simulink model "TST_AirCtl_Co"  (R2016b)
settings: Solver=FixedStepDiscrete  StartTime=0.0  StopTime=simTime  FixedStep=sampleTime  RelTol=1e-3
values from neighbouring files (symbols this model uses):
  testCase = 1    [initTST_AirCtl_Co_001.m]    (also in initTST_AirCtl_Co_002.m = 2)
libraries: simulink x19, UnitTest_Lib x16
settings Model: Creator=zhulinfeng  LastModifiedBy=zhulinfeng
settings DebuggingCC: SignalRangeChecking=error

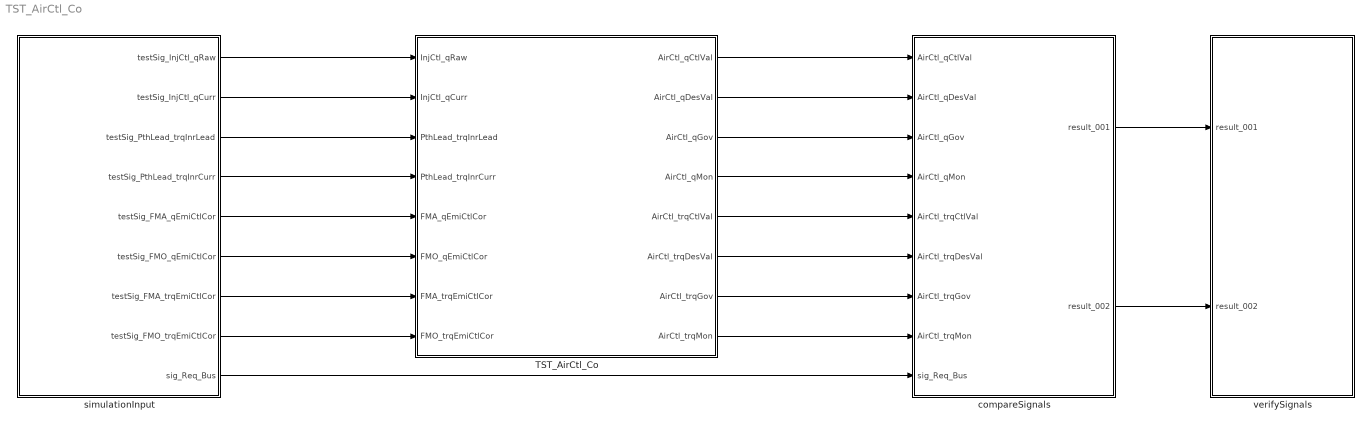
== system TST_AirCtl_Co ==
  TST_AirCtl_Co : Subsystem
  compareSignals : Subsystem
  simulationInput : Subsystem
  verifySignals : Subsystem
  wires:
  simulationInput/1(testSig_InjCtl_qRaw) -> TST_AirCtl_Co/1(InjCtl_qRaw)
  simulationInput/2(testSig_InjCtl_qCurr) -> TST_AirCtl_Co/2(InjCtl_qCurr)
  simulationInput/3(testSig_PthLead_trqInrLead) -> TST_AirCtl_Co/3(PthLead_trqInrLead)
  simulationInput/4(testSig_PthLead_trqInrCurr) -> TST_AirCtl_Co/4(PthLead_trqInrCurr)
  simulationInput/5(testSig_FMA_qEmiCtlCor) -> TST_AirCtl_Co/5(FMA_qEmiCtlCor)
  simulationInput/6(testSig_FMO_qEmiCtlCor) -> TST_AirCtl_Co/6(FMO_qEmiCtlCor)
  simulationInput/7(testSig_FMA_trqEmiCtlCor) -> TST_AirCtl_Co/7(FMA_trqEmiCtlCor)
  simulationInput/8(testSig_FMO_trqEmiCtlCor) -> TST_AirCtl_Co/8(FMO_trqEmiCtlCor)
  TST_AirCtl_Co/1(AirCtl_qCtlVal) -> compareSignals/1(AirCtl_qCtlVal)
  TST_AirCtl_Co/2(AirCtl_qDesVal) -> compareSignals/2(AirCtl_qDesVal)
  TST_AirCtl_Co/3(AirCtl_qGov) -> compareSignals/3(AirCtl_qGov)
  TST_AirCtl_Co/4(AirCtl_qMon) -> compareSignals/4(AirCtl_qMon)
  TST_AirCtl_Co/5(AirCtl_trqCtlVal) -> compareSignals/5(AirCtl_trqCtlVal)
  TST_AirCtl_Co/6(AirCtl_trqDesVal) -> compareSignals/6(AirCtl_trqDesVal)
  TST_AirCtl_Co/7(AirCtl_trqGov) -> compareSignals/7(AirCtl_trqGov)
  TST_AirCtl_Co/8(AirCtl_trqMon) -> compareSignals/8(AirCtl_trqMon)
  simulationInput/9(sig_Req_Bus) -> compareSignals/9(sig_Req_Bus)
  compareSignals/1(result_001) -> verifySignals/1(result_001)
  compareSignals/2(result_002) -> verifySignals/2(result_002)

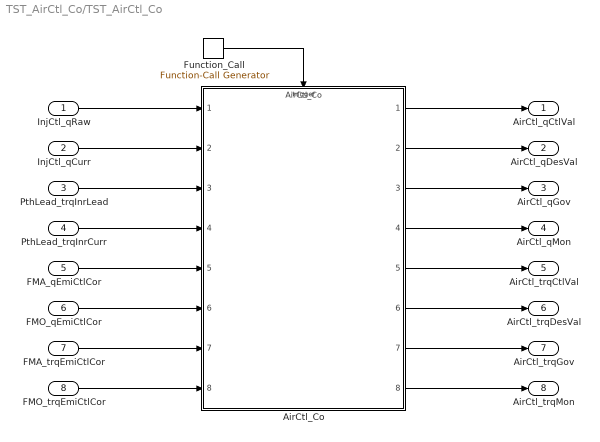
== system TST_AirCtl_Co/TST_AirCtl_Co ==
  InjCtl_qRaw : Inport
  InjCtl_qCurr : Inport  Port=2
  PthLead_trqInrLead : Inport  Port=3
  PthLead_trqInrCurr : Inport  Port=4
  FMA_qEmiCtlCor : Inport  Port=5
  FMO_qEmiCtlCor : Inport  Port=6
  FMA_trqEmiCtlCor : Inport  Port=7
  FMO_trqEmiCtlCor : Inport  Port=8
  AirCtl_Co : ModelReference  ModelNameDialog=AirCtl_Co  SimulationMode=Normal  ModelReferenceVersion=1.15  TriggerPortName=function  TriggerPortTriggerType=function-call  TriggerPortStatesWhenEnabling=held
  Function_Call : simulink/Ports & Subsystems/Function-Call Generator  sample_time=sampleTime  numberOfIterations=1
  AirCtl_qCtlVal : Outport
  AirCtl_qDesVal : Outport  Port=2
  AirCtl_qGov : Outport  Port=3
  AirCtl_qMon : Outport  Port=4
  AirCtl_trqCtlVal : Outport  Port=5
  AirCtl_trqDesVal : Outport  Port=6
  AirCtl_trqGov : Outport  Port=7
  AirCtl_trqMon : Outport  Port=8
  wires:
  Function_Call/1 -> AirCtl_Co/Trigger
  InjCtl_qRaw/1 -> AirCtl_Co/1
  InjCtl_qCurr/1 -> AirCtl_Co/2
  PthLead_trqInrLead/1 -> AirCtl_Co/3
  PthLead_trqInrCurr/1 -> AirCtl_Co/4
  FMA_qEmiCtlCor/1 -> AirCtl_Co/5
  FMO_qEmiCtlCor/1 -> AirCtl_Co/6
  FMA_trqEmiCtlCor/1 -> AirCtl_Co/7
  FMO_trqEmiCtlCor/1 -> AirCtl_Co/8
  AirCtl_Co/1 -> AirCtl_qCtlVal/1
  AirCtl_Co/2 -> AirCtl_qDesVal/1
  AirCtl_Co/3 -> AirCtl_qGov/1
  AirCtl_Co/4 -> AirCtl_qMon/1
  AirCtl_Co/5 -> AirCtl_trqCtlVal/1
  AirCtl_Co/6 -> AirCtl_trqDesVal/1
  AirCtl_Co/7 -> AirCtl_trqGov/1
  AirCtl_Co/8 -> AirCtl_trqMon/1

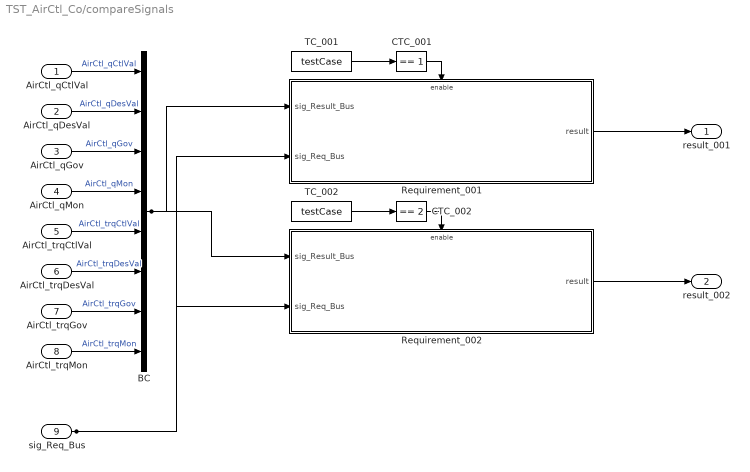
== system TST_AirCtl_Co/compareSignals ==
  AirCtl_qCtlVal : Inport
  AirCtl_qDesVal : Inport  Port=2
  AirCtl_qGov : Inport  Port=3
  AirCtl_qMon : Inport  Port=4
  AirCtl_trqCtlVal : Inport  Port=5
  AirCtl_trqDesVal : Inport  Port=6
  AirCtl_trqGov : Inport  Port=7
  AirCtl_trqMon : Inport  Port=8
  sig_Req_Bus : Inport  Port=9
  BC : BusCreator  Inputs=8
  CTC_001 : simulink/Logic and Bit Operations/Compare To Constant  relop===  const=1  OutDataTypeStr=boolean
  CTC_002 : simulink/Logic and Bit Operations/Compare To Constant  relop===  const=2  OutDataTypeStr=boolean
  Requirement_001 : Subsystem
  Requirement_002 : Subsystem
  TC_001 : Constant  Value=testCase
  TC_002 : Constant  Value=testCase
  result_001 : Outport
  result_002 : Outport  Port=2
  wires:
  AirCtl_qCtlVal/1 -> BC/1  "AirCtl_qCtlVal"
  AirCtl_qDesVal/1 -> BC/2  "AirCtl_qDesVal"
  AirCtl_qGov/1 -> BC/3  "AirCtl_qGov"
  AirCtl_qMon/1 -> BC/4  "AirCtl_qMon"
  AirCtl_trqCtlVal/1 -> BC/5  "AirCtl_trqCtlVal"
  AirCtl_trqDesVal/1 -> BC/6  "AirCtl_trqDesVal"
  AirCtl_trqGov/1 -> BC/7  "AirCtl_trqGov"
  AirCtl_trqMon/1 -> BC/8  "AirCtl_trqMon"
  TC_001/1 -> CTC_001/1
  CTC_001/1 -> Requirement_001/Enable
  sig_Req_Bus/1 -> Requirement_001/2(sig_Req_Bus), Requirement_002/2(sig_Req_Bus)
  BC/1 -> Requirement_001/1(sig_Result_Bus), Requirement_002/1(sig_Result_Bus)
  Requirement_001/1(result) -> result_001/1
  TC_002/1 -> CTC_002/1
  CTC_002/1 -> Requirement_002/Enable
  Requirement_002/1(result) -> result_002/1

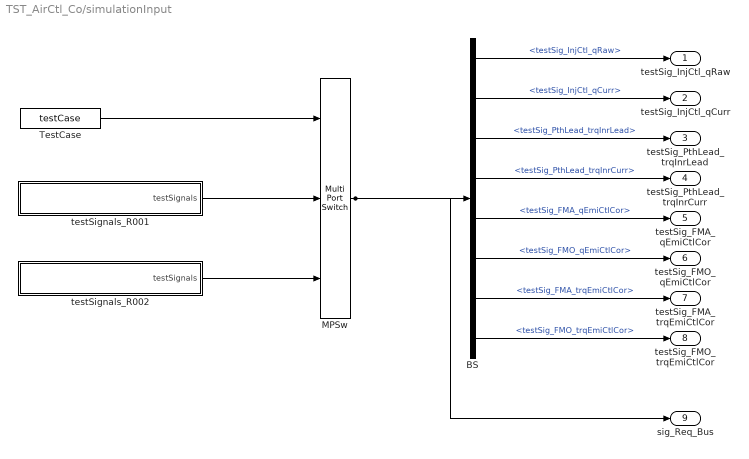
== system TST_AirCtl_Co/simulationInput ==
  BS : BusSelector  OutputSignals=testSig_InjCtl_qRaw,testSig_InjCtl_qCurr,testSig_PthLead_trqInrLead,testSig_PthLead_trqInrCurr,testSig_FMA_qEmiCtlCor,testSig_FMO_qEmiCtlCor,testSig_FMA_trqEmiCtlCor,testSig_FMO_trqEmiCtlCor
  MPSw : MultiPortSwitch  Inputs=2  SaturateOnIntegerOverflow=on  InputSameDT=on
  TestCase : Constant  Value=testCase
  testSignals_R001 : Subsystem
  testSignals_R002 : Subsystem
  testSig_InjCtl_qRaw : Outport
  testSig_InjCtl_qCurr : Outport  Port=2
  testSig_PthLead_trqInrLead : Outport  Port=3
  testSig_PthLead_trqInrCurr : Outport  Port=4
  testSig_FMA_qEmiCtlCor : Outport  Port=5
  testSig_FMO_qEmiCtlCor : Outport  Port=6
  testSig_FMA_trqEmiCtlCor : Outport  Port=7
  testSig_FMO_trqEmiCtlCor : Outport  Port=8
  sig_Req_Bus : Outport  Port=9
  wires:
  BS/1 -> testSig_InjCtl_qRaw/1  "<testSig_InjCtl_qRaw>"
  BS/2 -> testSig_InjCtl_qCurr/1  "<testSig_InjCtl_qCurr>"
  BS/3 -> testSig_PthLead_trqInrLead/1  "<testSig_PthLead_trqInrLead>"
  BS/4 -> testSig_PthLead_trqInrCurr/1  "<testSig_PthLead_trqInrCurr>"
  BS/5 -> testSig_FMA_qEmiCtlCor/1  "<testSig_FMA_qEmiCtlCor>"
  BS/6 -> testSig_FMO_qEmiCtlCor/1  "<testSig_FMO_qEmiCtlCor>"
  BS/7 -> testSig_FMA_trqEmiCtlCor/1  "<testSig_FMA_trqEmiCtlCor>"
  BS/8 -> testSig_FMO_trqEmiCtlCor/1  "<testSig_FMO_trqEmiCtlCor>"
  MPSw/1 -> BS/1, sig_Req_Bus/1
  TestCase/1 -> MPSw/1
  testSignals_R001/1(testSignals) -> MPSw/2
  testSignals_R002/1(testSignals) -> MPSw/3

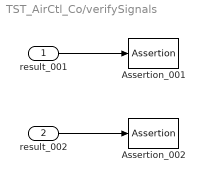
== system TST_AirCtl_Co/verifySignals ==
  result_001 : Inport
  result_002 : Inport  Port=2
  Assertion_001 : Assertion  Enabled=off
  Assertion_002 : Assertion  Enabled=off
  wires:
  result_001/1 -> Assertion_001/1
  result_002/1 -> Assertion_002/1

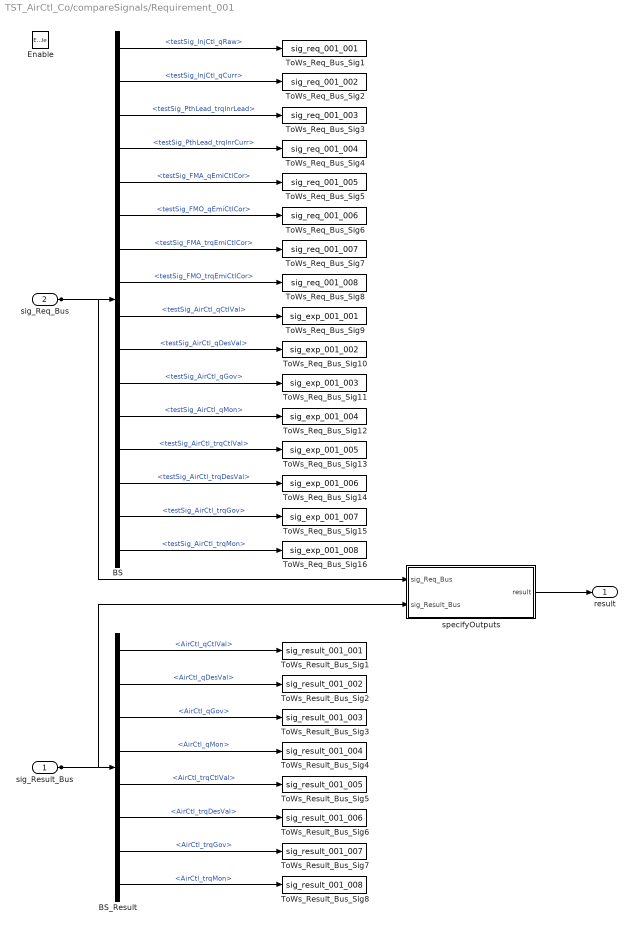
== system TST_AirCtl_Co/compareSignals/Requirement_001 ==
  sig_Result_Bus : Inport
  sig_Req_Bus : Inport  Port=2
  Enable : EnablePort
  BS : BusSelector  OutputSignals=testSig_InjCtl_qRaw,testSig_InjCtl_qCurr,testSig_PthLead_trqInrLead,testSig_PthLead_trqInrCurr,testSig_FMA_qEmiCtlCor,testSig_FMO_qEmiCtlCor,testSig_FMA_trqEmiCtlCor,testSig_FMO_trqEmiCtlCor,testSig_AirCtl_qCtlVal,testSig_AirCtl_qDesVal,testSig_AirCtl_qGov,testSig_AirCtl_qMon,testSig_AirCtl_trqCtlVal,testSig_AirCtl_trqDesVal,testSig_AirCtl_trqGov,testSig_AirCtl_trqMon
  BS_Result : BusSelector  OutputSignals=AirCtl_qCtlVal,AirCtl_qDesVal,AirCtl_qGov,AirCtl_qMon,AirCtl_trqCtlVal,AirCtl_trqDesVal,AirCtl_trqGov,AirCtl_trqMon
  ToWs_Req_Bus_Sig1 : ToWorkspace  VariableName=sig_req_001_001  SaveFormat=Structure With Time
  ToWs_Req_Bus_Sig10 : ToWorkspace  VariableName=sig_exp_001_002  SaveFormat=Structure With Time
  ToWs_Req_Bus_Sig11 : ToWorkspace  VariableName=sig_exp_001_003  SaveFormat=Structure With Time
  ToWs_Req_Bus_Sig12 : ToWorkspace  VariableName=sig_exp_001_004  SaveFormat=Structure With Time
  ToWs_Req_Bus_Sig13 : ToWorkspace  VariableName=sig_exp_001_005  SaveFormat=Structure With Time
  ToWs_Req_Bus_Sig14 : ToWorkspace  VariableName=sig_exp_001_006  SaveFormat=Structure With Time
  ToWs_Req_Bus_Sig15 : ToWorkspace  VariableName=sig_exp_001_007  SaveFormat=Structure With Time
  ToWs_Req_Bus_Sig16 : ToWorkspace  VariableName=sig_exp_001_008  SaveFormat=Structure With Time
  ToWs_Req_Bus_Sig2 : ToWorkspace  VariableName=sig_req_001_002  SaveFormat=Structure With Time
  ToWs_Req_Bus_Sig3 : ToWorkspace  VariableName=sig_req_001_003  SaveFormat=Structure With Time
  ToWs_Req_Bus_Sig4 : ToWorkspace  VariableName=sig_req_001_004  SaveFormat=Structure With Time
  ToWs_Req_Bus_Sig5 : ToWorkspace  VariableName=sig_req_001_005  SaveFormat=Structure With Time
  ToWs_Req_Bus_Sig6 : ToWorkspace  VariableName=sig_req_001_006  SaveFormat=Structure With Time
  ToWs_Req_Bus_Sig7 : ToWorkspace  VariableName=sig_req_001_007  SaveFormat=Structure With Time
  ToWs_Req_Bus_Sig8 : ToWorkspace  VariableName=sig_req_001_008  SaveFormat=Structure With Time
  ToWs_Req_Bus_Sig9 : ToWorkspace  VariableName=sig_exp_001_001  SaveFormat=Structure With Time
  ToWs_Result_Bus_Sig1 : ToWorkspace  VariableName=sig_result_001_001  SaveFormat=Structure With Time
  ToWs_Result_Bus_Sig2 : ToWorkspace  VariableName=sig_result_001_002  SaveFormat=Structure With Time
  ToWs_Result_Bus_Sig3 : ToWorkspace  VariableName=sig_result_001_003  SaveFormat=Structure With Time
  ToWs_Result_Bus_Sig4 : ToWorkspace  VariableName=sig_result_001_004  SaveFormat=Structure With Time
  ToWs_Result_Bus_Sig5 : ToWorkspace  VariableName=sig_result_001_005  SaveFormat=Structure With Time
  ToWs_Result_Bus_Sig6 : ToWorkspace  VariableName=sig_result_001_006  SaveFormat=Structure With Time
  ToWs_Result_Bus_Sig7 : ToWorkspace  VariableName=sig_result_001_007  SaveFormat=Structure With Time
  ToWs_Result_Bus_Sig8 : ToWorkspace  VariableName=sig_result_001_008  SaveFormat=Structure With Time
  specifyOutputs : Subsystem
  result : Outport
  wires:
  sig_Req_Bus/1 -> BS/1, specifyOutputs/1(sig_Req_Bus)
  BS/1 -> ToWs_Req_Bus_Sig1/1  "<testSig_InjCtl_qRaw>"
  BS/2 -> ToWs_Req_Bus_Sig2/1  "<testSig_InjCtl_qCurr>"
  BS/3 -> ToWs_Req_Bus_Sig3/1  "<testSig_PthLead_trqInrLead>"
  BS/4 -> ToWs_Req_Bus_Sig4/1  "<testSig_PthLead_trqInrCurr>"
  BS/5 -> ToWs_Req_Bus_Sig5/1  "<testSig_FMA_qEmiCtlCor>"
  BS/6 -> ToWs_Req_Bus_Sig6/1  "<testSig_FMO_qEmiCtlCor>"
  BS/7 -> ToWs_Req_Bus_Sig7/1  "<testSig_FMA_trqEmiCtlCor>"
  BS/8 -> ToWs_Req_Bus_Sig8/1  "<testSig_FMO_trqEmiCtlCor>"
  BS/9 -> ToWs_Req_Bus_Sig9/1  "<testSig_AirCtl_qCtlVal>"
  BS/10 -> ToWs_Req_Bus_Sig10/1  "<testSig_AirCtl_qDesVal>"
  BS/11 -> ToWs_Req_Bus_Sig11/1  "<testSig_AirCtl_qGov>"
  BS/12 -> ToWs_Req_Bus_Sig12/1  "<testSig_AirCtl_qMon>"
  BS/13 -> ToWs_Req_Bus_Sig13/1  "<testSig_AirCtl_trqCtlVal>"
  BS/14 -> ToWs_Req_Bus_Sig14/1  "<testSig_AirCtl_trqDesVal>"
  BS/15 -> ToWs_Req_Bus_Sig15/1  "<testSig_AirCtl_trqGov>"
  BS/16 -> ToWs_Req_Bus_Sig16/1  "<testSig_AirCtl_trqMon>"
  sig_Result_Bus/1 -> BS_Result/1, specifyOutputs/2(sig_Result_Bus)
  BS_Result/1 -> ToWs_Result_Bus_Sig1/1  "<AirCtl_qCtlVal>"
  BS_Result/2 -> ToWs_Result_Bus_Sig2/1  "<AirCtl_qDesVal>"
  BS_Result/3 -> ToWs_Result_Bus_Sig3/1  "<AirCtl_qGov>"
  BS_Result/4 -> ToWs_Result_Bus_Sig4/1  "<AirCtl_qMon>"
  BS_Result/5 -> ToWs_Result_Bus_Sig5/1  "<AirCtl_trqCtlVal>"
  BS_Result/6 -> ToWs_Result_Bus_Sig6/1  "<AirCtl_trqDesVal>"
  BS_Result/7 -> ToWs_Result_Bus_Sig7/1  "<AirCtl_trqGov>"
  BS_Result/8 -> ToWs_Result_Bus_Sig8/1  "<AirCtl_trqMon>"
  specifyOutputs/1(result) -> result/1

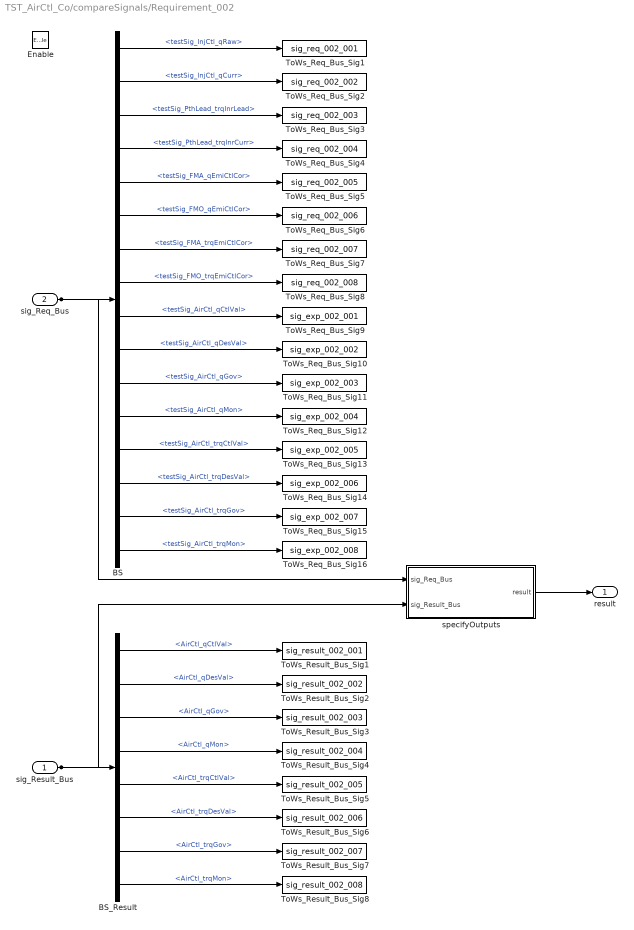
== system TST_AirCtl_Co/compareSignals/Requirement_002 ==
  sig_Result_Bus : Inport
  sig_Req_Bus : Inport  Port=2
  Enable : EnablePort
  BS : BusSelector  OutputSignals=testSig_InjCtl_qRaw,testSig_InjCtl_qCurr,testSig_PthLead_trqInrLead,testSig_PthLead_trqInrCurr,testSig_FMA_qEmiCtlCor,testSig_FMO_qEmiCtlCor,testSig_FMA_trqEmiCtlCor,testSig_FMO_trqEmiCtlCor,testSig_AirCtl_qCtlVal,testSig_AirCtl_qDesVal,testSig_AirCtl_qGov,testSig_AirCtl_qMon,testSig_AirCtl_trqCtlVal,testSig_AirCtl_trqDesVal,testSig_AirCtl_trqGov,testSig_AirCtl_trqMon
  BS_Result : BusSelector  OutputSignals=AirCtl_qCtlVal,AirCtl_qDesVal,AirCtl_qGov,AirCtl_qMon,AirCtl_trqCtlVal,AirCtl_trqDesVal,AirCtl_trqGov,AirCtl_trqMon
  ToWs_Req_Bus_Sig1 : ToWorkspace  VariableName=sig_req_002_001  SaveFormat=Structure With Time
  ToWs_Req_Bus_Sig10 : ToWorkspace  VariableName=sig_exp_002_002  SaveFormat=Structure With Time
  ToWs_Req_Bus_Sig11 : ToWorkspace  VariableName=sig_exp_002_003  SaveFormat=Structure With Time
  ToWs_Req_Bus_Sig12 : ToWorkspace  VariableName=sig_exp_002_004  SaveFormat=Structure With Time
  ToWs_Req_Bus_Sig13 : ToWorkspace  VariableName=sig_exp_002_005  SaveFormat=Structure With Time
  ToWs_Req_Bus_Sig14 : ToWorkspace  VariableName=sig_exp_002_006  SaveFormat=Structure With Time
  ToWs_Req_Bus_Sig15 : ToWorkspace  VariableName=sig_exp_002_007  SaveFormat=Structure With Time
  ToWs_Req_Bus_Sig16 : ToWorkspace  VariableName=sig_exp_002_008  SaveFormat=Structure With Time
  ToWs_Req_Bus_Sig2 : ToWorkspace  VariableName=sig_req_002_002  SaveFormat=Structure With Time
  ToWs_Req_Bus_Sig3 : ToWorkspace  VariableName=sig_req_002_003  SaveFormat=Structure With Time
  ToWs_Req_Bus_Sig4 : ToWorkspace  VariableName=sig_req_002_004  SaveFormat=Structure With Time
  ToWs_Req_Bus_Sig5 : ToWorkspace  VariableName=sig_req_002_005  SaveFormat=Structure With Time
  ToWs_Req_Bus_Sig6 : ToWorkspace  VariableName=sig_req_002_006  SaveFormat=Structure With Time
  ToWs_Req_Bus_Sig7 : ToWorkspace  VariableName=sig_req_002_007  SaveFormat=Structure With Time
  ToWs_Req_Bus_Sig8 : ToWorkspace  VariableName=sig_req_002_008  SaveFormat=Structure With Time
  ToWs_Req_Bus_Sig9 : ToWorkspace  VariableName=sig_exp_002_001  SaveFormat=Structure With Time
  ToWs_Result_Bus_Sig1 : ToWorkspace  VariableName=sig_result_002_001  SaveFormat=Structure With Time
  ToWs_Result_Bus_Sig2 : ToWorkspace  VariableName=sig_result_002_002  SaveFormat=Structure With Time
  ToWs_Result_Bus_Sig3 : ToWorkspace  VariableName=sig_result_002_003  SaveFormat=Structure With Time
  ToWs_Result_Bus_Sig4 : ToWorkspace  VariableName=sig_result_002_004  SaveFormat=Structure With Time
  ToWs_Result_Bus_Sig5 : ToWorkspace  VariableName=sig_result_002_005  SaveFormat=Structure With Time
  ToWs_Result_Bus_Sig6 : ToWorkspace  VariableName=sig_result_002_006  SaveFormat=Structure With Time
  ToWs_Result_Bus_Sig7 : ToWorkspace  VariableName=sig_result_002_007  SaveFormat=Structure With Time
  ToWs_Result_Bus_Sig8 : ToWorkspace  VariableName=sig_result_002_008  SaveFormat=Structure With Time
  specifyOutputs : Subsystem
  result : Outport
  wires:
  sig_Req_Bus/1 -> BS/1, specifyOutputs/1(sig_Req_Bus)
  BS/1 -> ToWs_Req_Bus_Sig1/1  "<testSig_InjCtl_qRaw>"
  BS/2 -> ToWs_Req_Bus_Sig2/1  "<testSig_InjCtl_qCurr>"
  BS/3 -> ToWs_Req_Bus_Sig3/1  "<testSig_PthLead_trqInrLead>"
  BS/4 -> ToWs_Req_Bus_Sig4/1  "<testSig_PthLead_trqInrCurr>"
  BS/5 -> ToWs_Req_Bus_Sig5/1  "<testSig_FMA_qEmiCtlCor>"
  BS/6 -> ToWs_Req_Bus_Sig6/1  "<testSig_FMO_qEmiCtlCor>"
  BS/7 -> ToWs_Req_Bus_Sig7/1  "<testSig_FMA_trqEmiCtlCor>"
  BS/8 -> ToWs_Req_Bus_Sig8/1  "<testSig_FMO_trqEmiCtlCor>"
  BS/9 -> ToWs_Req_Bus_Sig9/1  "<testSig_AirCtl_qCtlVal>"
  BS/10 -> ToWs_Req_Bus_Sig10/1  "<testSig_AirCtl_qDesVal>"
  BS/11 -> ToWs_Req_Bus_Sig11/1  "<testSig_AirCtl_qGov>"
  BS/12 -> ToWs_Req_Bus_Sig12/1  "<testSig_AirCtl_qMon>"
  BS/13 -> ToWs_Req_Bus_Sig13/1  "<testSig_AirCtl_trqCtlVal>"
  BS/14 -> ToWs_Req_Bus_Sig14/1  "<testSig_AirCtl_trqDesVal>"
  BS/15 -> ToWs_Req_Bus_Sig15/1  "<testSig_AirCtl_trqGov>"
  BS/16 -> ToWs_Req_Bus_Sig16/1  "<testSig_AirCtl_trqMon>"
  sig_Result_Bus/1 -> BS_Result/1, specifyOutputs/2(sig_Result_Bus)
  BS_Result/1 -> ToWs_Result_Bus_Sig1/1  "<AirCtl_qCtlVal>"
  BS_Result/2 -> ToWs_Result_Bus_Sig2/1  "<AirCtl_qDesVal>"
  BS_Result/3 -> ToWs_Result_Bus_Sig3/1  "<AirCtl_qGov>"
  BS_Result/4 -> ToWs_Result_Bus_Sig4/1  "<AirCtl_qMon>"
  BS_Result/5 -> ToWs_Result_Bus_Sig5/1  "<AirCtl_trqCtlVal>"
  BS_Result/6 -> ToWs_Result_Bus_Sig6/1  "<AirCtl_trqDesVal>"
  BS_Result/7 -> ToWs_Result_Bus_Sig7/1  "<AirCtl_trqGov>"
  BS_Result/8 -> ToWs_Result_Bus_Sig8/1  "<AirCtl_trqMon>"
  specifyOutputs/1(result) -> result/1

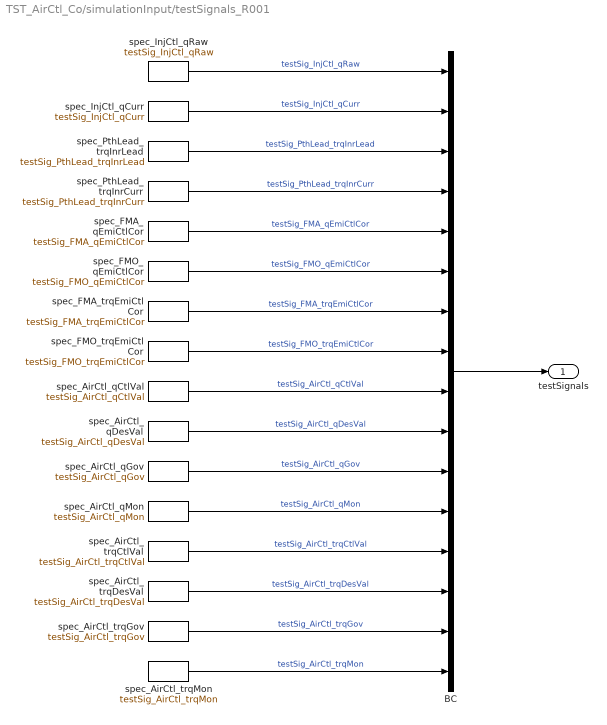
== system TST_AirCtl_Co/simulationInput/testSignals_R001 ==
  BC : BusCreator  Inputs=16
  spec_AirCtl_qCtlVal : FromWorkspace  VariableName=testSig_AirCtl_qCtlVal  Interpolate=off  OutputAfterFinalValue=Holding final value
  spec_AirCtl_qDesVal : FromWorkspace  VariableName=testSig_AirCtl_qDesVal  Interpolate=off  OutputAfterFinalValue=Holding final value
  spec_AirCtl_qGov : FromWorkspace  VariableName=testSig_AirCtl_qGov  Interpolate=off  OutputAfterFinalValue=Holding final value
  spec_AirCtl_qMon : FromWorkspace  VariableName=testSig_AirCtl_qMon  Interpolate=off  OutputAfterFinalValue=Holding final value
  spec_AirCtl_trqCtlVal : FromWorkspace  VariableName=testSig_AirCtl_trqCtlVal  Interpolate=off  OutputAfterFinalValue=Holding final value
  spec_AirCtl_trqDesVal : FromWorkspace  VariableName=testSig_AirCtl_trqDesVal  Interpolate=off  OutputAfterFinalValue=Holding final value
  spec_AirCtl_trqGov : FromWorkspace  VariableName=testSig_AirCtl_trqGov  Interpolate=off  OutputAfterFinalValue=Holding final value
  spec_AirCtl_trqMon : FromWorkspace  VariableName=testSig_AirCtl_trqMon  Interpolate=off  OutputAfterFinalValue=Holding final value
  spec_FMA_qEmiCtlCor : FromWorkspace  VariableName=testSig_FMA_qEmiCtlCor  Interpolate=off  OutputAfterFinalValue=Holding final value
  spec_FMA_trqEmiCtlCor : FromWorkspace  VariableName=testSig_FMA_trqEmiCtlCor  Interpolate=off  OutputAfterFinalValue=Holding final value
  spec_FMO_qEmiCtlCor : FromWorkspace  VariableName=testSig_FMO_qEmiCtlCor  Interpolate=off  OutputAfterFinalValue=Holding final value
  spec_FMO_trqEmiCtlCor : FromWorkspace  VariableName=testSig_FMO_trqEmiCtlCor  Interpolate=off  OutputAfterFinalValue=Holding final value
  spec_InjCtl_qCurr : FromWorkspace  VariableName=testSig_InjCtl_qCurr  Interpolate=off  OutputAfterFinalValue=Holding final value
  spec_InjCtl_qRaw : FromWorkspace  VariableName=testSig_InjCtl_qRaw  Interpolate=off  OutputAfterFinalValue=Holding final value
  spec_PthLead_trqInrCurr : FromWorkspace  VariableName=testSig_PthLead_trqInrCurr  Interpolate=off  OutputAfterFinalValue=Holding final value
  spec_PthLead_trqInrLead : FromWorkspace  VariableName=testSig_PthLead_trqInrLead  Interpolate=off  OutputAfterFinalValue=Holding final value
  testSignals : Outport
  wires:
  BC/1 -> testSignals/1
  spec_InjCtl_qRaw/1 -> BC/1  "testSig_InjCtl_qRaw"
  spec_InjCtl_qCurr/1 -> BC/2  "testSig_InjCtl_qCurr"
  spec_PthLead_trqInrLead/1 -> BC/3  "testSig_PthLead_trqInrLead"
  spec_PthLead_trqInrCurr/1 -> BC/4  "testSig_PthLead_trqInrCurr"
  spec_FMA_qEmiCtlCor/1 -> BC/5  "testSig_FMA_qEmiCtlCor"
  spec_FMO_qEmiCtlCor/1 -> BC/6  "testSig_FMO_qEmiCtlCor"
  spec_FMA_trqEmiCtlCor/1 -> BC/7  "testSig_FMA_trqEmiCtlCor"
  spec_FMO_trqEmiCtlCor/1 -> BC/8  "testSig_FMO_trqEmiCtlCor"
  spec_AirCtl_qCtlVal/1 -> BC/9  "testSig_AirCtl_qCtlVal"
  spec_AirCtl_qDesVal/1 -> BC/10  "testSig_AirCtl_qDesVal"
  spec_AirCtl_qGov/1 -> BC/11  "testSig_AirCtl_qGov"
  spec_AirCtl_qMon/1 -> BC/12  "testSig_AirCtl_qMon"
  spec_AirCtl_trqCtlVal/1 -> BC/13  "testSig_AirCtl_trqCtlVal"
  spec_AirCtl_trqDesVal/1 -> BC/14  "testSig_AirCtl_trqDesVal"
  spec_AirCtl_trqGov/1 -> BC/15  "testSig_AirCtl_trqGov"
  spec_AirCtl_trqMon/1 -> BC/16  "testSig_AirCtl_trqMon"

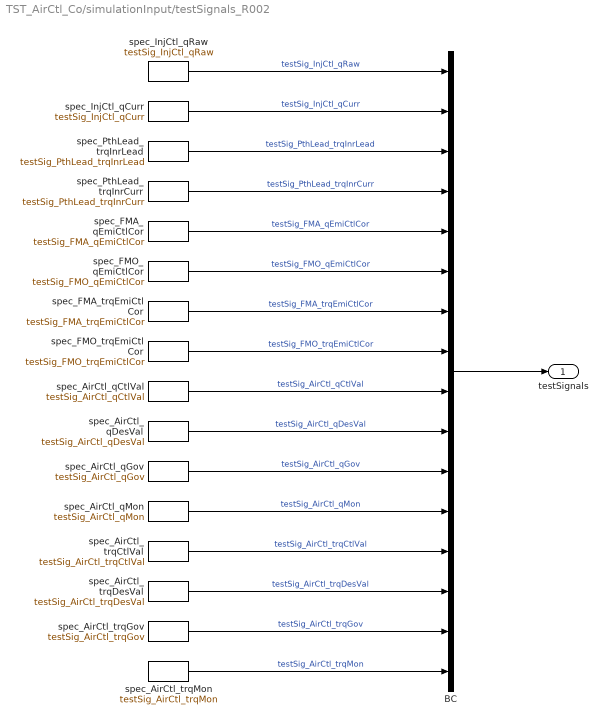
== system TST_AirCtl_Co/simulationInput/testSignals_R002 ==
  BC : BusCreator  Inputs=16
  spec_AirCtl_qCtlVal : FromWorkspace  VariableName=testSig_AirCtl_qCtlVal  Interpolate=off  OutputAfterFinalValue=Holding final value
  spec_AirCtl_qDesVal : FromWorkspace  VariableName=testSig_AirCtl_qDesVal  Interpolate=off  OutputAfterFinalValue=Holding final value
  spec_AirCtl_qGov : FromWorkspace  VariableName=testSig_AirCtl_qGov  Interpolate=off  OutputAfterFinalValue=Holding final value
  spec_AirCtl_qMon : FromWorkspace  VariableName=testSig_AirCtl_qMon  Interpolate=off  OutputAfterFinalValue=Holding final value
  spec_AirCtl_trqCtlVal : FromWorkspace  VariableName=testSig_AirCtl_trqCtlVal  Interpolate=off  OutputAfterFinalValue=Holding final value
  spec_AirCtl_trqDesVal : FromWorkspace  VariableName=testSig_AirCtl_trqDesVal  Interpolate=off  OutputAfterFinalValue=Holding final value
  spec_AirCtl_trqGov : FromWorkspace  VariableName=testSig_AirCtl_trqGov  Interpolate=off  OutputAfterFinalValue=Holding final value
  spec_AirCtl_trqMon : FromWorkspace  VariableName=testSig_AirCtl_trqMon  Interpolate=off  OutputAfterFinalValue=Holding final value
  spec_FMA_qEmiCtlCor : FromWorkspace  VariableName=testSig_FMA_qEmiCtlCor  Interpolate=off  OutputAfterFinalValue=Holding final value
  spec_FMA_trqEmiCtlCor : FromWorkspace  VariableName=testSig_FMA_trqEmiCtlCor  Interpolate=off  OutputAfterFinalValue=Holding final value
  spec_FMO_qEmiCtlCor : FromWorkspace  VariableName=testSig_FMO_qEmiCtlCor  Interpolate=off  OutputAfterFinalValue=Holding final value
  spec_FMO_trqEmiCtlCor : FromWorkspace  VariableName=testSig_FMO_trqEmiCtlCor  Interpolate=off  OutputAfterFinalValue=Holding final value
  spec_InjCtl_qCurr : FromWorkspace  VariableName=testSig_InjCtl_qCurr  Interpolate=off  OutputAfterFinalValue=Holding final value
  spec_InjCtl_qRaw : FromWorkspace  VariableName=testSig_InjCtl_qRaw  Interpolate=off  OutputAfterFinalValue=Holding final value
  spec_PthLead_trqInrCurr : FromWorkspace  VariableName=testSig_PthLead_trqInrCurr  Interpolate=off  OutputAfterFinalValue=Holding final value
  spec_PthLead_trqInrLead : FromWorkspace  VariableName=testSig_PthLead_trqInrLead  Interpolate=off  OutputAfterFinalValue=Holding final value
  testSignals : Outport
  wires:
  BC/1 -> testSignals/1
  spec_InjCtl_qRaw/1 -> BC/1  "testSig_InjCtl_qRaw"
  spec_InjCtl_qCurr/1 -> BC/2  "testSig_InjCtl_qCurr"
  spec_PthLead_trqInrLead/1 -> BC/3  "testSig_PthLead_trqInrLead"
  spec_PthLead_trqInrCurr/1 -> BC/4  "testSig_PthLead_trqInrCurr"
  spec_FMA_qEmiCtlCor/1 -> BC/5  "testSig_FMA_qEmiCtlCor"
  spec_FMO_qEmiCtlCor/1 -> BC/6  "testSig_FMO_qEmiCtlCor"
  spec_FMA_trqEmiCtlCor/1 -> BC/7  "testSig_FMA_trqEmiCtlCor"
  spec_FMO_trqEmiCtlCor/1 -> BC/8  "testSig_FMO_trqEmiCtlCor"
  spec_AirCtl_qCtlVal/1 -> BC/9  "testSig_AirCtl_qCtlVal"
  spec_AirCtl_qDesVal/1 -> BC/10  "testSig_AirCtl_qDesVal"
  spec_AirCtl_qGov/1 -> BC/11  "testSig_AirCtl_qGov"
  spec_AirCtl_qMon/1 -> BC/12  "testSig_AirCtl_qMon"
  spec_AirCtl_trqCtlVal/1 -> BC/13  "testSig_AirCtl_trqCtlVal"
  spec_AirCtl_trqDesVal/1 -> BC/14  "testSig_AirCtl_trqDesVal"
  spec_AirCtl_trqGov/1 -> BC/15  "testSig_AirCtl_trqGov"
  spec_AirCtl_trqMon/1 -> BC/16  "testSig_AirCtl_trqMon"

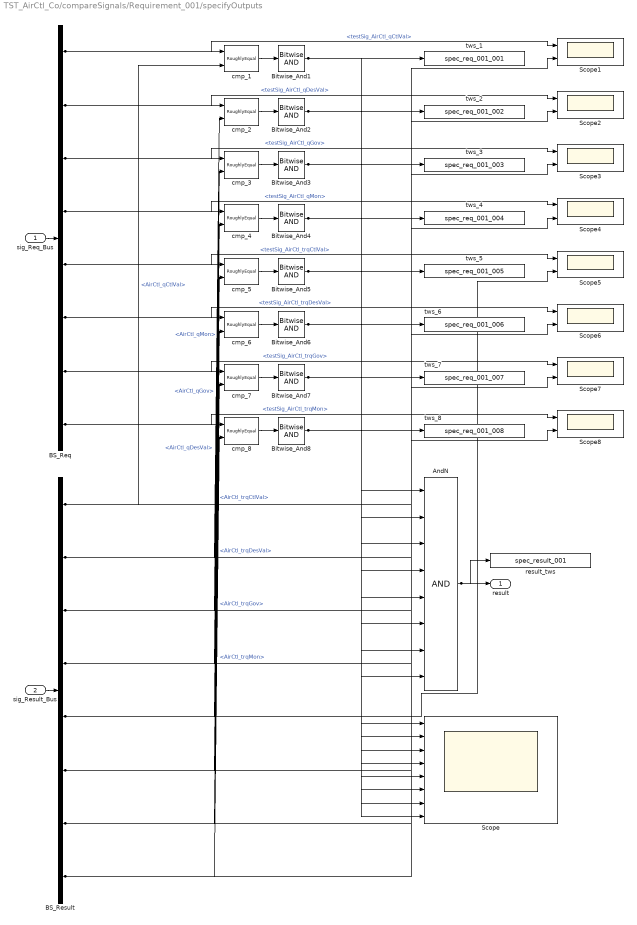
== system TST_AirCtl_Co/compareSignals/Requirement_001/specifyOutputs ==
  sig_Req_Bus : Inport
  sig_Result_Bus : Inport  Port=2
  AndN : Logic  Inputs=8
  BS_Req : BusSelector  OutputSignals=testSig_AirCtl_qCtlVal,testSig_AirCtl_qDesVal,testSig_AirCtl_qGov,testSig_AirCtl_qMon,testSig_AirCtl_trqCtlVal,testSig_AirCtl_trqDesVal,testSig_AirCtl_trqGov,testSig_AirCtl_trqMon
  BS_Result : BusSelector  OutputSignals=AirCtl_qCtlVal,AirCtl_qDesVal,AirCtl_qGov,AirCtl_qMon,AirCtl_trqCtlVal,AirCtl_trqDesVal,AirCtl_trqGov,AirCtl_trqMon
  Bitwise_And{1..8} (8 alike) : simulink/Logic and Bit Operations/Bitwise Operator  logicop=AND  UseBitMask=off  BitMask=bin2dec('11011001')  BitMaskRealWorld=Stored Integer
  Scope : Scope  NumInputPorts=8
  Scope{1..8} (8 alike) : Scope  NumInputPorts=2
  cmp_{1..8} (8 alike) : UnitTest_Lib/RoughlyEqual  slope=0.1
  result_tws : ToWorkspace  VariableName=spec_result_001
  tws_1 : ToWorkspace  VariableName=spec_req_001_001
  tws_2 : ToWorkspace  VariableName=spec_req_001_002
  tws_3 : ToWorkspace  VariableName=spec_req_001_003
  tws_4 : ToWorkspace  VariableName=spec_req_001_004
  tws_5 : ToWorkspace  VariableName=spec_req_001_005
  tws_6 : ToWorkspace  VariableName=spec_req_001_006
  tws_7 : ToWorkspace  VariableName=spec_req_001_007
  tws_8 : ToWorkspace  VariableName=spec_req_001_008
  result : Outport
  wires:
  sig_Req_Bus/1 -> BS_Req/1
  sig_Result_Bus/1 -> BS_Result/1
  AndN/1 -> result/1, result_tws/1
  BS_Req/1 -> cmp_1/1, Scope1/1  "<testSig_AirCtl_qCtlVal>"
  BS_Result/1 -> cmp_1/2, Scope1/2  "<AirCtl_qCtlVal>"
  cmp_1/1 -> Bitwise_And1/1
  Bitwise_And1/1 -> tws_1/1, AndN/1, Scope/1
  BS_Req/2 -> cmp_2/1, Scope2/1  "<testSig_AirCtl_qDesVal>"
  BS_Result/2 -> cmp_2/2, Scope2/2  "<AirCtl_qDesVal>"
  cmp_2/1 -> Bitwise_And2/1
  Bitwise_And2/1 -> tws_2/1, AndN/2, Scope/2
  BS_Req/3 -> cmp_3/1, Scope3/1  "<testSig_AirCtl_qGov>"
  BS_Result/3 -> cmp_3/2, Scope3/2  "<AirCtl_qGov>"
  cmp_3/1 -> Bitwise_And3/1
  Bitwise_And3/1 -> tws_3/1, AndN/3, Scope/3
  BS_Req/4 -> cmp_4/1, Scope4/1  "<testSig_AirCtl_qMon>"
  BS_Result/4 -> cmp_4/2, Scope4/2  "<AirCtl_qMon>"
  cmp_4/1 -> Bitwise_And4/1
  Bitwise_And4/1 -> tws_4/1, AndN/4, Scope/4
  BS_Req/5 -> cmp_5/1, Scope5/1  "<testSig_AirCtl_trqCtlVal>"
  BS_Result/5 -> cmp_5/2, Scope5/2  "<AirCtl_trqCtlVal>"
  cmp_5/1 -> Bitwise_And5/1
  Bitwise_And5/1 -> tws_5/1, AndN/5, Scope/5
  BS_Req/6 -> cmp_6/1, Scope6/1  "<testSig_AirCtl_trqDesVal>"
  BS_Result/6 -> cmp_6/2, Scope6/2  "<AirCtl_trqDesVal>"
  cmp_6/1 -> Bitwise_And6/1
  Bitwise_And6/1 -> tws_6/1, AndN/6, Scope/6
  BS_Req/7 -> cmp_7/1, Scope7/1  "<testSig_AirCtl_trqGov>"
  BS_Result/7 -> cmp_7/2, Scope7/2  "<AirCtl_trqGov>"
  cmp_7/1 -> Bitwise_And7/1
  Bitwise_And7/1 -> tws_7/1, AndN/7, Scope/7
  BS_Req/8 -> cmp_8/1, Scope8/1  "<testSig_AirCtl_trqMon>"
  BS_Result/8 -> cmp_8/2, Scope8/2  "<AirCtl_trqMon>"
  cmp_8/1 -> Bitwise_And8/1
  Bitwise_And8/1 -> tws_8/1, AndN/8, Scope/8

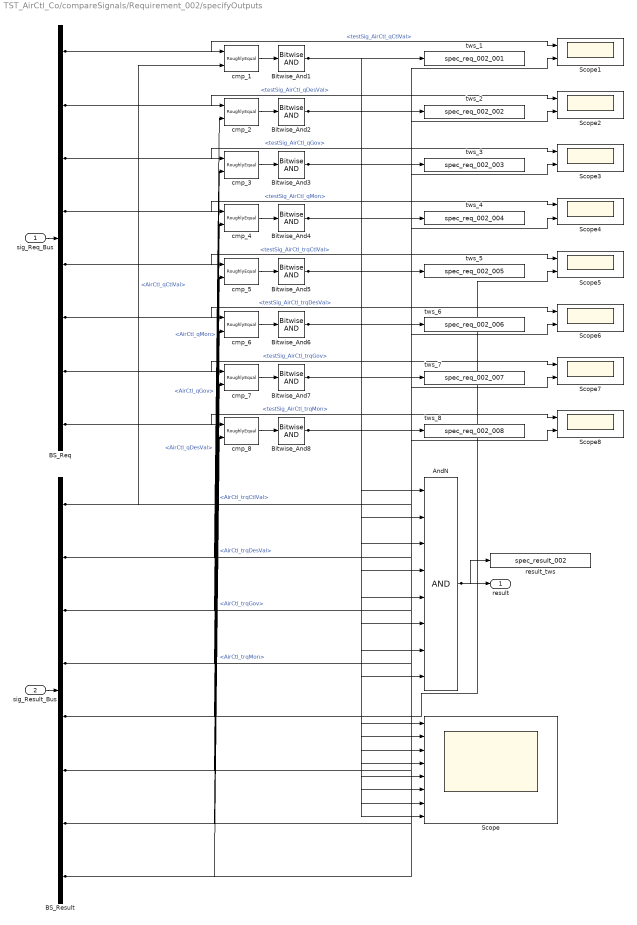
== system TST_AirCtl_Co/compareSignals/Requirement_002/specifyOutputs ==
  sig_Req_Bus : Inport
  sig_Result_Bus : Inport  Port=2
  AndN : Logic  Inputs=8
  BS_Req : BusSelector  OutputSignals=testSig_AirCtl_qCtlVal,testSig_AirCtl_qDesVal,testSig_AirCtl_qGov,testSig_AirCtl_qMon,testSig_AirCtl_trqCtlVal,testSig_AirCtl_trqDesVal,testSig_AirCtl_trqGov,testSig_AirCtl_trqMon
  BS_Result : BusSelector  OutputSignals=AirCtl_qCtlVal,AirCtl_qDesVal,AirCtl_qGov,AirCtl_qMon,AirCtl_trqCtlVal,AirCtl_trqDesVal,AirCtl_trqGov,AirCtl_trqMon
  Bitwise_And{1..8} (8 alike) : simulink/Logic and Bit Operations/Bitwise Operator  logicop=AND  UseBitMask=off  BitMask=bin2dec('11011001')  BitMaskRealWorld=Stored Integer
  Scope : Scope  NumInputPorts=8
  Scope{1..8} (8 alike) : Scope  NumInputPorts=2
  cmp_{1..8} (8 alike) : UnitTest_Lib/RoughlyEqual  slope=0.1
  result_tws : ToWorkspace  VariableName=spec_result_002
  tws_1 : ToWorkspace  VariableName=spec_req_002_001
  tws_2 : ToWorkspace  VariableName=spec_req_002_002
  tws_3 : ToWorkspace  VariableName=spec_req_002_003
  tws_4 : ToWorkspace  VariableName=spec_req_002_004
  tws_5 : ToWorkspace  VariableName=spec_req_002_005
  tws_6 : ToWorkspace  VariableName=spec_req_002_006
  tws_7 : ToWorkspace  VariableName=spec_req_002_007
  tws_8 : ToWorkspace  VariableName=spec_req_002_008
  result : Outport
  wires:
  sig_Req_Bus/1 -> BS_Req/1
  sig_Result_Bus/1 -> BS_Result/1
  AndN/1 -> result/1, result_tws/1
  BS_Req/1 -> cmp_1/1, Scope1/1  "<testSig_AirCtl_qCtlVal>"
  BS_Result/1 -> cmp_1/2, Scope1/2  "<AirCtl_qCtlVal>"
  cmp_1/1 -> Bitwise_And1/1
  Bitwise_And1/1 -> tws_1/1, AndN/1, Scope/1
  BS_Req/2 -> cmp_2/1, Scope2/1  "<testSig_AirCtl_qDesVal>"
  BS_Result/2 -> cmp_2/2, Scope2/2  "<AirCtl_qDesVal>"
  cmp_2/1 -> Bitwise_And2/1
  Bitwise_And2/1 -> tws_2/1, AndN/2, Scope/2
  BS_Req/3 -> cmp_3/1, Scope3/1  "<testSig_AirCtl_qGov>"
  BS_Result/3 -> cmp_3/2, Scope3/2  "<AirCtl_qGov>"
  cmp_3/1 -> Bitwise_And3/1
  Bitwise_And3/1 -> tws_3/1, AndN/3, Scope/3
  BS_Req/4 -> cmp_4/1, Scope4/1  "<testSig_AirCtl_qMon>"
  BS_Result/4 -> cmp_4/2, Scope4/2  "<AirCtl_qMon>"
  cmp_4/1 -> Bitwise_And4/1
  Bitwise_And4/1 -> tws_4/1, AndN/4, Scope/4
  BS_Req/5 -> cmp_5/1, Scope5/1  "<testSig_AirCtl_trqCtlVal>"
  BS_Result/5 -> cmp_5/2, Scope5/2  "<AirCtl_trqCtlVal>"
  cmp_5/1 -> Bitwise_And5/1
  Bitwise_And5/1 -> tws_5/1, AndN/5, Scope/5
  BS_Req/6 -> cmp_6/1, Scope6/1  "<testSig_AirCtl_trqDesVal>"
  BS_Result/6 -> cmp_6/2, Scope6/2  "<AirCtl_trqDesVal>"
  cmp_6/1 -> Bitwise_And6/1
  Bitwise_And6/1 -> tws_6/1, AndN/6, Scope/6
  BS_Req/7 -> cmp_7/1, Scope7/1  "<testSig_AirCtl_trqGov>"
  BS_Result/7 -> cmp_7/2, Scope7/2  "<AirCtl_trqGov>"
  cmp_7/1 -> Bitwise_And7/1
  Bitwise_And7/1 -> tws_7/1, AndN/7, Scope/7
  BS_Req/8 -> cmp_8/1, Scope8/1  "<testSig_AirCtl_trqMon>"
  BS_Result/8 -> cmp_8/2, Scope8/2  "<AirCtl_trqMon>"
  cmp_8/1 -> Bitwise_And8/1
  Bitwise_And8/1 -> tws_8/1, AndN/8, Scope/8
